simulink model "Racing_2019"  (R2017a)
settings: Solver=FixedStepDiscrete  StartTime=0.0  StopTime=Inf  FixedStep=1e-3  RelTol=1e-3  EnableMultiTasking=on
PostLoadFcn:
  | , if any(exist('dsrtsu_mdlpostloadfcn', 'file') == [2, 3, 6]), try dsrtsu_mdlpostloadfcn('Execute', bdroot); catch fprintf('Error in PostLoadFcn (dsrtsu_mdlpostloadfcn) for model "%s":\n %s\n', bdroot, lasterr); end, end,
undefined symbols (not defined in the file): Accu_Fans_Enable, Accu_Fans_ON, Accu_Fans_PWM, APPS_Bypass, APPS_Value, AUX_Error_Time, Batt_Temp_High_Threshold, Batt_Temp_Low_Threshold, BMS_Error_Time, BMS_Reset, BMS_Reset_Enable, BMS_Status_Bypass, Brake_Plausibility_Threshold, Brake_Threshold, Brakelight_Test, Braking_Torque, BSPD_State_Bypass, Buzzer, Buzzer_Silent, Buzzer_Test, Calibrate, CAN_Rx_FMEA_Enable, CAN_Status_FMEA_Enable, CAN_Tx_FMEA_Enable, Car_Reset, Car_Reset_Enable, Dash_Fan_PWM, DiscIntNeverNeededParam, DRS_Enable, DRS_PWM_OFF, DRS_PWM_ON, ED_Enable, ED_On, Eject_USB, Enable_Kill, Enable_LED_Test, Fans_Left_Enable, Fans_Left_ON, Fans_Left_PWM, Fans_Right_Enable, Fans_Right_ON, Fans_Right_PWM, I_MAX, IGBT_Temp_High_Threshold, IGBT_Temp_Low_Threshold, Inverter_CAN_Tx_Enable, Inverter_Frequency, KW_Max_Regen_Reset, KW_Max_Reset, LV_DCDC_Temp_High_Threshold, LV_DCDC_Temp_Low_Threshold, magnitude, Plausibility_Bypass, Power_Limiter_Killswitch, Power_Target_kW, Pump_Left_Enable, Pump_Left_ON, Pump_Right_Enable, Pump_Right_ON, Pump_Signal_Left ... (+13)
libraries: rtiusbflightreclib x206, simulink x153, rtican x52, powerlib_meascontrol x47, simulink_extras x17, rti1401lib_adc_type4 x6, rti1401lib_dio_type4 x3, rti1401lib_II_base x1
(part 23 of 23)

== matlab function Racing_2019/Accu CAN Rx/Segment 5/s5t1 ==
  data: x input; y output
function y = thermBMS(x)
y = (1/(0.003354016+0.000256524*log(((10000*x)/(5-x))/10000)+0.00000260597*(log(((10000*x)/(5-x))/100000))*(log(((10000*x)/(5-x))/10000))+0.0000000632926*(log(((100000*x)/(5-x))/10000))*(log(((10000*x)/(5-x))/10000))*(log(((10000*x)/(5-x))/10000))))-273.15
end

== matlab function Racing_2019/Accu CAN Rx/Segment 5/s5t2 ==
  data: x input; y output
function y = thermBMS(x)
y = (1/(0.003354016+0.000256524*log(((10000*x)/(5-x))/10000)+0.00000260597*(log(((10000*x)/(5-x))/100000))*(log(((10000*x)/(5-x))/10000))+0.0000000632926*(log(((100000*x)/(5-x))/10000))*(log(((10000*x)/(5-x))/10000))*(log(((10000*x)/(5-x))/10000))))-273.15
end

== matlab function Racing_2019/Accu CAN Rx/Segment 5/s5t3 ==
  data: x input; y output
function y = thermBMS(x)
y = (1/(0.003354016+0.000256524*log(((10000*x)/(5-x))/10000)+0.00000260597*(log(((10000*x)/(5-x))/100000))*(log(((10000*x)/(5-x))/10000))+0.0000000632926*(log(((100000*x)/(5-x))/10000))*(log(((10000*x)/(5-x))/10000))*(log(((10000*x)/(5-x))/10000))))-273.15
end

== matlab function Racing_2019/Accu CAN Rx/Segment 5/s5t4 ==
  data: x input; y output
function y = thermBMS(x)
y = (1/(0.003354016+0.000256524*log(((10000*x)/(5-x))/10000)+0.00000260597*(log(((10000*x)/(5-(x*0.0015)))/100000))*(log(((10000*x)/(5-x))/10000))+0.0000000632926*(log(((100000*x)/(5-x))/10000))*(log(((10000*x)/(5-x))/10000))*(log(((10000*x)/(5-x))/10000))))-273.15
end

== matlab function Racing_2019/Accu CAN Rx/Segment 6/s6t1 ==
  data: x input; y output
function y = thermBMS(x)
y = (1/(0.003354016+0.000256524*log(((10000*x)/(5-x))/10000)+0.00000260597*(log(((10000*x)/(5-x))/100000))*(log(((10000*x)/(5-x))/10000))+0.0000000632926*(log(((100000*x)/(5-x))/10000))*(log(((10000*x)/(5-x))/10000))*(log(((10000*x)/(5-x))/10000))))-273.15
end

== matlab function Racing_2019/Accu CAN Rx/Segment 6/s6t2 ==
  data: x input; y output
function y = thermBMS(x)
y = (1/(0.003354016+0.000256524*log(((10000*x)/(5-x))/10000)+0.00000260597*(log(((10000*x)/(5-x))/100000))*(log(((10000*x)/(5-x))/10000))+0.0000000632926*(log(((100000*x)/(5-x))/10000))*(log(((10000*x)/(5-x))/10000))*(log(((10000*x)/(5-x))/10000))))-273.15
end

== matlab function Racing_2019/Accu CAN Rx/Segment 6/s6t3 ==
  data: x input; y output
function y = thermBMS(x)
y = (1/(0.003354016+0.000256524*log(((10000*x)/(5-x))/10000)+0.00000260597*(log(((10000*x)/(5-x))/100000))*(log(((10000*x)/(5-x))/10000))+0.0000000632926*(log(((100000*x)/(5-x))/10000))*(log(((10000*x)/(5-x))/10000))*(log(((10000*x)/(5-x))/10000))))-273.15
end

== matlab function Racing_2019/Accu CAN Rx/Segment 6/s6t4 ==
  data: x input; y output
function y = thermBMS(x)
y = (1/(0.003354016+0.000256524*log(((10000*x)/(5-x))/10000)+0.00000260597*(log(((10000*x)/(5-(x*0.0015)))/100000))*(log(((10000*x)/(5-x))/10000))+0.0000000632926*(log(((100000*x)/(5-x))/10000))*(log(((10000*x)/(5-x))/10000))*(log(((10000*x)/(5-x))/10000))))-273.15
end

== matlab function Racing_2019/Accu CAN Rx/Segment 7/s7t1 ==
  data: x input; y output
function y = thermBMS(x)
y = (1/(0.003354016+0.000256524*log(((10000*x)/(5-x))/10000)+0.00000260597*(log(((10000*x)/(5-x))/100000))*(log(((10000*x)/(5-x))/10000))+0.0000000632926*(log(((100000*x)/(5-x))/10000))*(log(((10000*x)/(5-x))/10000))*(log(((10000*x)/(5-x))/10000))))-272.15
end

== matlab function Racing_2019/Accu CAN Rx/Segment 7/s7t2 ==
  data: x input; y output
function y = thermBMS(x)
y = (1/(0.003354016+0.000256524*log(((10000*x)/(5-x))/10000)+0.00000260597*(log(((10000*x)/(5-x))/100000))*(log(((10000*x)/(5-x))/10000))+0.0000000632926*(log(((100000*x)/(5-x))/10000))*(log(((10000*x)/(5-x))/10000))*(log(((10000*x)/(5-x))/10000))))-272.15
end

== matlab function Racing_2019/Accu CAN Rx/Segment 7/s7t3 ==
  data: x input; y output
function y = thermBMS(x)
y = (1/(0.003354016+0.000256524*log(((10000*x)/(5-x))/10000)+0.00000260597*(log(((10000*x)/(5-x))/100000))*(log(((10000*x)/(5-x))/10000))+0.0000000632926*(log(((100000*x)/(5-x))/10000))*(log(((10000*x)/(5-x))/10000))*(log(((10000*x)/(5-x))/10000))))-272.15
end

== matlab function Racing_2019/Accu CAN Rx/Segment 7/s7t4 ==
  data: x input; y output
function y = thermBMS(x)
y = (1/(0.003354016+0.000256524*log(((10000*x)/(5-x))/10000)+0.00000260597*(log(((10000*x)/(5-(x*0.0015)))/100000))*(log(((10000*x)/(5-x))/10000))+0.0000000632926*(log(((100000*x)/(5-x))/10000))*(log(((10000*x)/(5-x))/10000))*(log(((10000*x)/(5-x))/10000))))-272.15
end

== matlab function Racing_2019/Inverters CAN Tx/Inverters CAN Send ==
  data: Mode output; ID output; i input; Icont input; Time output; RPMmax input
function [Mode,ID,Time] = fcn(i,Icont,RPMmax)

Icont10 = Icont * 10;
IcontHex = dec2hex(Icont10);
IcontHexFinal = '000';

if Icont < 26
    IcontHexFinal(1:1) = '0';
    IcontHexFinal(2:3) = IcontHex;
    IcontLhex = IcontHexFinal(2:3);
    IcontHhex = IcontHexFinal(1:1);
    IcontL = hex2dec(IcontLhex);
    IcontH = hex2dec(IcontHhex);
else
    IcontHexFinal = IcontHex;
    IcontLhex = IcontHexFinal(2:3);
    IcontHhex = IcontHexFinal(1:1);
    IcontL = hex2dec(IcontLhex);
    IcontH = hex2dec(IcontHhex);
end

RPM_max = RPMmax;
RPM_maxHex = dec2hex(RPM_max);
RPM_maxHexFinal = '000';

if RPM_max < 26
    RPM_maxHexFinal(1:1) = '0';
    RPM_maxHexFinal(2:3) = IcontHex;
    RPM_maxLhex = RPM_maxHexFinal(2:3);
    RPM_maxHhex = RPM_maxHexFinal(1:1);
    RPM_maxL = hex2dec(RPM_maxLhex);
    RPM_maxH = hex2dec(RPM_maxHhex);
else
    RPM_maxHexFinal = RPM_maxHex;
    RPM_maxLhex = RPM_maxHexFinal(2:3);
    RPM_maxHhex = RPM_maxHexFinal(1:1);
    RPM_maxL = hex2dec(RPM_maxLhex);
    RPM_maxH = hex2dec(RPM_maxHhex);
end

%Start-Up Information
%I_Max
if i==-14
    Mode=61;
    ID=77;
    Time=0;
%I_Contiuous
elseif i==-13
    Mode=61;
    ID=78;
    Time=0;
%RPM_Max
elseif i==-12
    Mode=61;
    ID=200;
    Time=0;
%I_Max
elseif i==-11
    Mode=61;
    ID=77;
    Time=0;
%I_Contiuous
elseif i==-10
    Mode=61;
    ID=78;
    Time=0;
%RPM_Max
elseif i==-9
    Mode=61;
    ID=200;
    Time=0;
%I_Max
elseif i==-8
    Mode=61;
    ID=77;
    Time=0;
%I_Contiuous
elseif i==-7
    Mode=61;
    ID=78;
    Time=0;
%RPM_Max
elseif i==-6
    Mode=61;
    ID=200;
    Time=0;
%I_Max
elseif i==-5
    Mode=61;
    ID=77;
    Time=0;
%I_Contiuous
elseif i==-4
    Mode=61;
    ID=78;
    Time=0;
%RPM_Max
elseif i==-3
    Mode=61;
    ID=200;
    Time=0;
%I_Max
elseif i==-2
    Mode=61;
    ID=77;
    Time=0;
%I_Contiuous
elseif i==-1
    Mode=61;
    ID=78;
    Time=0;
%RPM_Max
elseif i==0
    Mode=61;
    ID=200;
    Time=0;
    

%RPM
elseif i==1
	Mode=61;
	ID=48;
	Time=10;
%Motor_Temp
elseif i==2
	Mode=61;
	ID=73;
	Time=250;
%Commanded_Torque
elseif i==3
	Mode=61;
	ID=34;
	Time=250;
%BTB
elseif i==4
	Mode=61;
	ID=226;
	Time=250;
%IGBT_Temp
elseif i==5
	Mode=61;
	ID=74;
	Time=250;
%Vout               
elseif i==6
	Mode=61;
    ID=138;           
	Time=250;
%I_Rms
elseif i==7
	Mode=61;
	ID=32;
	Time=10;
%Error
elseif i==8
	Mode=61;
	ID=143;
	Time=250;
%RPM
elseif i==9
	Mode=61;
	ID=48;
	Time=10;
%Motor_Temp
elseif i==10
	Mode=61;
	ID=73;
	Time=100;
%Commanded_Torque
elseif i==11
	Mode=61;
	ID=34;
	Time=250;
%BTB
elseif i==12
	Mode=61;
	ID=226;
	Time=250;
%IGBT_Temp
elseif i==13
	Mode=61;
	ID=74;
	Time=250;
%Vout               
elseif i==14
	Mode=61;
    ID=138;           
	Time=250;
%I_Rms
elseif i==15
	Mode=61;
	ID=32;
	Time=10;
%Error
elseif i==16
	Mode=61;
	ID=143;
	Time=250;
%I_MAX
elseif i==17
	Mode=61;
	ID=77;
	Time=0;
%I_Continuous
elseif i==18
	Mode=61;
	ID=78;
	Time=0;
%RPM_Max
elseif i==19
	Mode=61;
	ID=200;
	Time=0;
    
    
%RPM
elseif i==101
	Mode=61;
	ID=48;
	Time=255;
%Motor_Temp
elseif i==102
	Mode=61;
	ID=73;
	Time=255;
%Commanded_Torque
elseif i==103
	Mode=61;
	ID=34;
	Time=255;
%BTB
elseif i==104
	Mode=61;
	ID=226;
	Time=255;
%IGBT_Temp
elseif i==105
	Mode=61;
	ID=74;
	Time=255;
%Vout               
elseif i==106
	Mode=61;
    ID=138;           
	Time=255;
%I_Rms
elseif i==107
	Mode=61;
	ID=32;
	Time=255;
%Error
elseif i==108
	Mode=61;
	ID=143;
	Time=255;

%Ask rpmMAX
elseif i==201   
    Mode=61;
    ID=200;
    Time=0;
%Ask I_Max
elseif i==202   
    Mode=61;
    ID=77;
    Time=0;
%Ask IContinuous
elseif i==203   
    Mode=61;
    ID=78;
    Time=0;

%Set Ipeak
elseif i==301   
    Mode=77;    %RegID
    ID=IcontL;    
    Time=IcontH; 
%Set Icont
elseif i==302   
    Mode=78;    %RegID
    ID=IcontL;     
    Time=IcontH;     

elseif i==401   %Write to EEPROM
    Mode=132;   %RegID for EEPROM write function
    ID=0;
    Time=0;
elseif i==501   %Read from EEPROM
    Mode=131;   %RegID for EEPROM read function
    ID=0;
    Time=0;
    
%Set RPM Limit
elseif i==601
    Mode=200;
    ID=RPM_maxL;
    Time=RPM_maxH;
    
else
    Mode=144;
    ID=0;
    Time=0;
end
end

== matlab function Racing_2019/The Journey of Torque/Power Limiter v3 (open-loop)/Irms Initialization ==
  data: Irms_Out output; Irms_In input
function Irms_Out  = fcn(Irms_In)

if Irms_In > 0
    Irms_Out = Irms_In;
else
    Irms_Out = 0;
end
end
